simulink model "pade1"  (Simulink 8.1)
settings: Solver=ode4  StartTime=0.0  StopTime=5.0  FixedStep=0.01  RelTol=1e-3
values from neighbouring files (symbols this model uses):
  k = 1    [pade1.mat]
  T = 1    [pade1.mat]
  tau = 2    [pade1.mat]    (also in pade2.mat = 0.966912085986; pade2_errc.m = x0(3))
settings Model: Creator=student  LastModifiedBy=adasdeb
settings DebuggingCC: FcnCallInpInsideContextMsg=EnableAllAsWarning
settings GRTTargetCC: CombineOutputUpdateFcns=on  GRTInterface=off

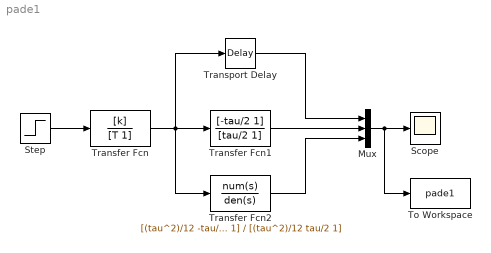
== system pade1 ==
  Mux : Mux  Inputs=3
  Scope : Scope
  Step : Step  Time=0  SampleTime=0
  To Workspace : ToWorkspace  VariableName=pade1  SampleTime=-1
  Transfer Fcn : TransferFcn  Numerator=[k]  Denominator=[T 1]
  Transfer Fcn1 : TransferFcn  Numerator=[-tau/2 1]  Denominator=[tau/2 1]
  Transfer Fcn2 : TransferFcn  Numerator=[(tau^2)/12 -tau/2 1]  Denominator=[(tau^2)/12 tau/2 1]
  Transport Delay : TransportDelay  DelayTime=tau
  wires:
  Step/1 -> Transfer Fcn/1
  Transfer Fcn/1 -> Transfer Fcn2/1, Transport Delay/1, Transfer Fcn1/1
  Transport Delay/1 -> Mux/1
  Transfer Fcn1/1 -> Mux/2
  Transfer Fcn2/1 -> Mux/3
  Mux/1 -> To Workspace/1, Scope/1
